simulink model "microgrid_ESS"  (R2023a)
settings: Solver=FixedStepDiscrete  StartTime=0.0  StopTime=90  FixedStep=Ts  RelTol=1e-3
PreLoadFcn:
  | %bus_ini
InitFcn:
  | %sim_param_ini
values from neighbouring files (symbols this model uses):
  Ts = 5.0E-5    [microgrid_system.sldd]
  Ts_PLC = 0.001    [microgrid_system.sldd]
undefined symbols (not defined in the file or in its folder): C, getfullname
libraries: microgridLib x37, slrealtimeutilitieslib x16, simulink x7, spsThreePhaseVIMeasurementLib x3, speedgoatlib_obsolete x3, spsPower3phInstantaneousLib x2, speedgoatlib_shared x1, spsThreePhaseSourceLib x1, spsThreePhaseFaultLib x1, spspowerguiLib x1, slrealtimetgmanagement x1
settings Model: DataDictionary=microgrid_system.sldd  SimulationMode=external  ExtModeEnableFloating=off  Creator=jlesage  LastModifiedBy=steve.liu
settings SolverCC: ConcurrentTasks=on  AlgebraicLoopSolver=TrustRegion  PositivePriorityOrder=on  AutoInsertRateTranBlk=on
settings OptimizationCC: BlockReduction=off  OptimizeBlockIOStorage=off  ReuseModelBlockBuffer=off
settings DebuggingCC: TasksWithSamePriorityMsg=none  UnconnectedInputMsg=warning  UnconnectedOutputMsg=warning  UnconnectedLineMsg=warning
settings HardwareCC: ProdBitPerLong=64  ProdLongLongMode=on  ProdHWDeviceType=Intel->x86-64 (Linux 64)
settings ModelReferenceCC: EnableRefExpFcnMdlSchedulingChecks=on
settings RTWCC: Description=Simulink Real-Time  SystemTargetFile=slrealtime.tlc  TemplateMakefile=slrealtime_default_tmf  Toolchain=Simulink Real-Time Toolchain  BuildConfiguration=Faster Runs  CodeExecutionProfiling=on  TargetLang=C++  DLArmComputeVersion=19.05

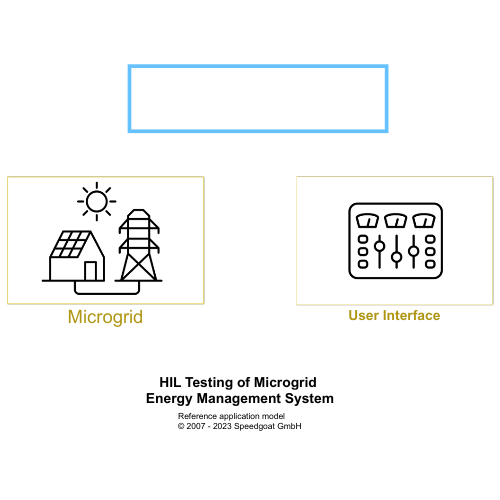
[thumbnail: Simulink's stored preview of the top-level diagram]
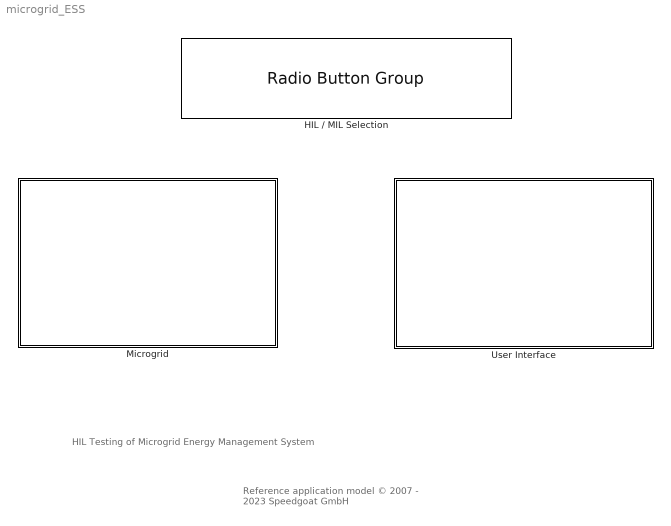
== system microgrid_ESS ==
  note: Reference application model
      | © 2007 - 2023 Speedgoat GmbH
  note: HIL Testing of Microgrid
      | Energy Management System
  HIL / MIL Selection : RadioButtonGroup  LabelPosition=Hide  SelectedLabel=Model-in-the-Loop (Desktop and real-time simulation)  ButtonGroupName=Simulation Mode
      settings: Values={{'Model-in-the-Loop (Desktop and real-time simulation)', 'Hardware-in-the-Loop'}, [0 1]}
  Microgrid : Subsystem
      mask Display: image('$imagefile'); % Use "Edit Image" on toolstrip to change.
  User Interface : Subsystem
      mask Display: image('$imagefile'); % Use "Edit Image" on toolstrip to change.

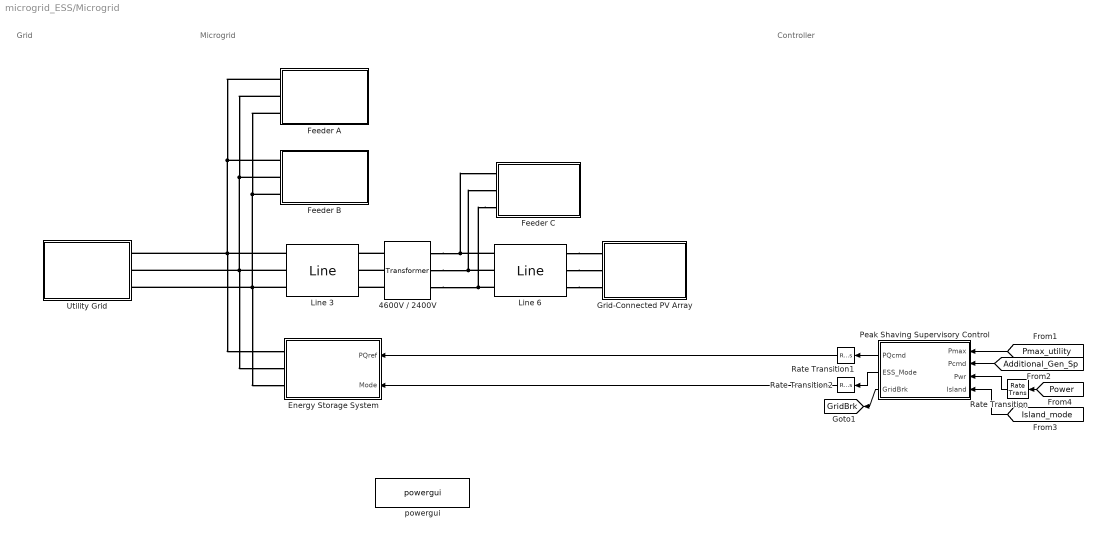
== system microgrid_ESS/Microgrid ==
  note: Microgrid
  note: Grid
  note: Controller
  4600V / 2400V : microgridLib/Transformer  kS=5000  Freq=60  Vp=4600  Vs=2400  Zperc=6.37  Ratio=3.5
  Energy Storage System : Subsystem
      settings: PortSchema="{\"entries\":[{\"content\":{\"sides\":[{\"content\":{\"connectorIds\":[\"LConn1\",\"LConn2\",\"LConn3\"]},\"type\":\"ConnectorPlacement.EquallySpacedRectSide\",\"uuid\":\"2732472e-ca9c-424c-87bd-53552b4deef9\"},{\"content\":{\"connectorIds\":[\"In1\",\"In2\"],\"side\":\"RIGHT\"},\"type\":\"ConnectorPlacement.EquallySpacedRectSide\",\"uuid\":\"774380c0-3a16-4d8f-bf4d-db561b2973b7\"},{\"content\":{\"connectorIds\":[],\"side\":\"TOP\"},\"type\":\"ConnectorPlacement.EquallySpacedRectSide\",\"uuid\":\"18303f45-8657-48d2-ba54-46513b679fcd\"}]},\"type\":\"ConnectorPlacement.EquallySpacedConnector\",\"uuid\":\"7e47473e-856d-4ee6-aecb-5fd96cc13303\"}],\"packageUris\":[\"http://schema.mathworks.com/mf0/Connector/R2020b\"],\"version\":\"1.0\"}"
      mask Display: image('$imagefile'); % Use "Edit Image" on toolstrip to change.
  Feeder A : Subsystem
      mask Display: image('$imagefile'); % Use "Edit Image" on toolstrip to change.
  Feeder B : Subsystem
      mask Display: image('$imagefile'); % Use "Edit Image" on toolstrip to change.
  Feeder C : Subsystem
      mask Display: image('$imagefile'); % Use "Edit Image" on toolstrip to change.
  Grid-Connected PV Array : Subsystem
      mask Display: image('$imagefile'); % Use "Edit Image" on toolstrip to change.
  Line 3 : microgridLib/Line   gauge=500 Kcmil  Freq=60  Length_ft=300  Ratio=3
  Line 6 : microgridLib/Line   gauge=4/0 AWG  Freq=60  Length_ft=25  Ratio=3
  Peak Shaving Supervisory Control : Subsystem  Variant=on
      mask Display: image('$imagefile'); % Use "Edit Image" on toolstrip to change.
  Rate Transition : RateTransition  OutPortSampleTime=Ts_PLC
  Rate Transition1 : RateTransition  OutPortSampleTime=Ts_Control
  Rate Transition2 : RateTransition  OutPortSampleTime=Ts_Control
  Utility Grid : Subsystem
      mask Display: image('$imagefile'); % Use "Edit Image" on toolstrip to change.
  powergui : spspowerguiLib/powergui  Priority=2  SimulationMode=Discrete  SampleTime=Ts  frequency=60  Iterations=50  frequencyindice=0  Pbase=1e6  ErrMax=0.0001  UnitsV=kV  UnitsW=MW  buscounter=6  FunctionMessages=off  echomessages=off  EnableUseOfTLC=off  CurrentSourceSwitches=off  DisableSnubberDevices=off  DisableRonSwitches=off  DisableVfSwitches=off  DisplayEquations=off  AutomaticDiscreteSolvers=off  SolverType=Tustin/Backward Euler (TBE)  Interpol=off  ExternalGateDelay=off  methode=off  Ts=0  x0status=blocks  SPID=off  SwTol=0  HookPort=off  NonlinearTolerance=1e-4  nMaxIteration=100  ContinueOnMaxIteration=off  RestoreLinks=warning  ResistiveCurrentMeasurement=off  Frange=logspace(0,3,50)  Ylog=off  Xlog=off  ShowGrid=off  save=off  variable=ZData  structure=0  ZoomFFT=on  StartTime=0.0  cycles=2  DisplayStyle=off  fundamental=60  FreqAxis=off  MaxFrequency=1000  frequencyindicesteady=1  RmsSteady=1  display=off
  tag scope: GridBrk=global
  wires:
  [Pmax_utility] -> Peak Shaving Supervisory Control/1(Pmax)
  [Additional_Gen_Sp] -> Peak Shaving Supervisory Control/2(Pcmd)
  Peak Shaving Supervisory Control/1(PQcmd) -> Rate Transition1/1
  [Island_mode] -> Peak Shaving Supervisory Control/4(Island)
  Rate Transition/1 -> Peak Shaving Supervisory Control/3(Pwr)
  Peak Shaving Supervisory Control/3(GridBrk) -> [GridBrk]
  [Power] -> Rate Transition/1
  Peak Shaving Supervisory Control/2(ESS_Mode) -> Rate Transition2/1
  Rate Transition1/1 -> Energy Storage System/1(PQref)
  Rate Transition2/1 -> Energy Storage System/2(Mode)
  connections:
  4600V / 2400V/LConn3 -- Line 3/RConn3
  Feeder C/LConn3 -- 4600V / 2400V/RConn3 -- Line 6/LConn3
  4600V / 2400V/LConn2 -- Line 3/RConn2
  Line 6/LConn2 -- 4600V / 2400V/RConn2 -- Feeder C/LConn2
  4600V / 2400V/LConn1 -- Line 3/RConn1
  Line 6/LConn1 -- 4600V / 2400V/RConn1 -- Feeder C/LConn1
  Line 3/LConn1 -- Feeder A/LConn1 -- Feeder B/LConn1 -- Utility Grid/RConn1 -- Energy Storage System/LConn1
  Line 3/LConn3 -- Feeder A/LConn3 -- Feeder B/LConn3 -- Utility Grid/RConn3 -- Energy Storage System/LConn3
  Feeder B/LConn2 -- Feeder A/LConn2 -- Utility Grid/RConn2 -- Energy Storage System/LConn2 -- Line 3/LConn2
  Line 6/RConn1 -- Grid-Connected PV Array/LConn1
  Line 6/RConn2 -- Grid-Connected PV Array/LConn2
  Line 6/RConn3 -- Grid-Connected PV Array/LConn3

== system microgrid_ESS/User Interface ==
  note: Power [W]
  note: Microgrid Peak-Shaving Control
  note: Additional Battery
      | Supply [MW]
  note: Utility Max Power
      | Setpoint [MW]
  note: Current
      | [A]
  Dashboard Scope : DashboardScope  TimeSpan=90  Ymin=-1e6  Ymax=1.5e6  ScaleAtStop=off
  Dashboard Scope1 : DashboardScope  TimeSpan=90  Ymin=-100  Ymax=100  ScaleAtStop=off
  Instrumentation : Subsystem
      mask Display: image('$imagefile'); % Use "Edit Image" on toolstrip to change.
  Knob : KnobBlock  ScaleMax=3
  Knob1 : KnobBlock  ScaleMin=-3  ScaleMax=3
  Toggle Switch : ToggleSwitchBlock  LabelPosition=Hide
      settings: Values={{'Grid Connect', 'Island'}, [0 1]}
  Toggle Switch1 : ToggleSwitchBlock  LabelPosition=Hide
      settings: Values={{'Clear', 'Cloud'}, [0 1]}

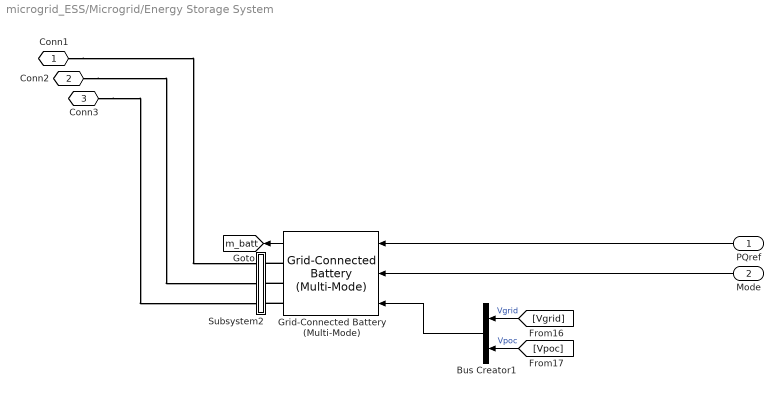
== system microgrid_ESS/Microgrid/Energy Storage System ==
  PQref : Inport
  Mode : Inport  Port=2
  Bus Creator1 : BusCreator  Inputs=2
  Grid-Connected Battery (Multi-Mode) : microgridLib/Grid-Connected Battery (Multi-Mode)  Pmod=25  Vnom_dc=480  Bcap=500  Vnom_prim=4600  Fnom=60  Ts=Ts  Ts_Control=Ts_Control
  Subsystem2 : Subsystem
  Conn1 : PMIOPort  Side=Left
  Conn2 : PMIOPort  Port=2  Side=Left
  Conn3 : PMIOPort  Port=3  Side=Left
  tag scope: m_batt=global
  wires:
  Bus Creator1/1 -> Grid-Connected Battery (Multi-Mode)/3
  Grid-Connected Battery (Multi-Mode)/1 -> [m_batt]
  [Vgrid] -> Bus Creator1/1  "Vgrid"
  [Vpoc] -> Bus Creator1/2  "Vpoc"
  PQref/1 -> Grid-Connected Battery (Multi-Mode)/1
  Mode/1 -> Grid-Connected Battery (Multi-Mode)/2
  connections:
  Grid-Connected Battery (Multi-Mode)/RConn2 -- Subsystem2/RConn2
  Grid-Connected Battery (Multi-Mode)/RConn3 -- Subsystem2/RConn3
  Grid-Connected Battery (Multi-Mode)/RConn1 -- Subsystem2/RConn1
  Conn2/RConn1 -- Subsystem2/LConn2
  Conn3/RConn1 -- Subsystem2/LConn3
  Conn1/RConn1 -- Subsystem2/LConn1

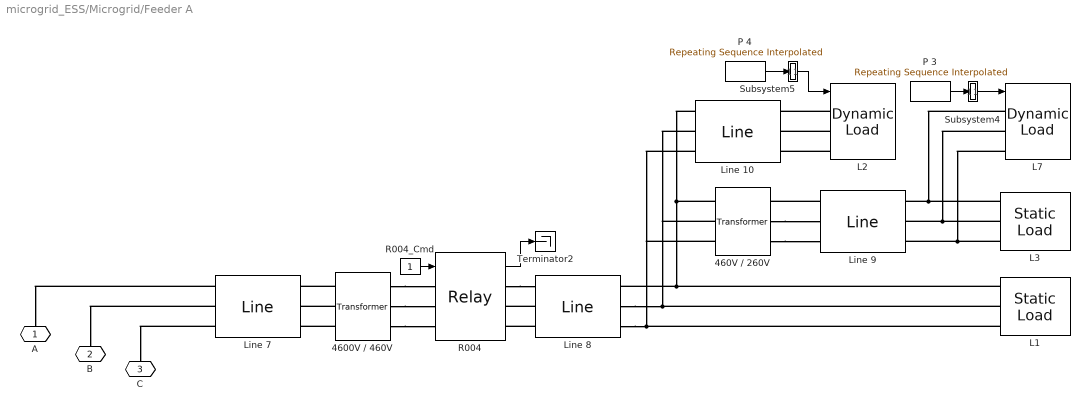
== system microgrid_ESS/Microgrid/Feeder A ==
  4600V / 460V : microgridLib/Transformer  kS=5000  Freq=60  Vp=4600  Vs=460  Zperc=5.1  Ratio=2.5
  460V / 260V : microgridLib/Transformer  kS=2000  Freq=60  Vp=460  Vs=240  Zperc=5.1  Ratio=2.5
  L1 : microgridLib/Static Load  kS=25  PF=0.9  Vrms=460  Freq=60
  L2 : microgridLib/Dynamic Load  Vrms=460  Freq=60  Ts=Ts  Tau=1e-4
  L3 : microgridLib/Static Load  kS=25  PF=1  Vrms=240  Freq=60
  L7 : microgridLib/Dynamic Load  Vrms=240  Freq=60  Ts=Ts  Tau=1e-4
  Line 10 : microgridLib/Line   gauge=3/0 AWG  Freq=60  Length_ft=50  Ratio=3
  Line 7 : microgridLib/Line   gauge=500 Kcmil  Freq=60  Length_ft=500  Ratio=3
  Line 8 : microgridLib/Line   gauge=500 Kcmil  Freq=60  Length_ft=100  Ratio=3
  Line 9 : microgridLib/Line   gauge=1/0 AWG  Freq=60  Length_ft=25  Ratio=3
  P 3 : simulink/Sources/Repeating Sequence Interpolated  OutValues=[0 -1e5 3e5 10e5 0e5 5e5 0]'/50  TimeValues=[0 5 10 25 30 45 60]'*0.2  LookUpMeth=Interpolation-Use End Values  tsamp=Ts  OutMin=[]  OutMax=[]  OutDataTypeStr=double  OutputDataTypeScalingMode=double  OutDataType=fixdt(0,8)  OutScaling=2^-10
  P 4 : simulink/Sources/Repeating Sequence Interpolated  OutValues=[0 1e5 -3e5 10e5 0e5 5e5 0]'/75  TimeValues=[0 5 10 25 30 45 60]'*0.5  LookUpMeth=Interpolation-Use End Values  tsamp=Ts  OutMin=[]  OutMax=[]  OutDataTypeStr=double  OutputDataTypeScalingMode=double  OutDataType=fixdt(0,8)  OutScaling=2^-10
  R004 : microgridLib/Relay  SystemSampleTime=-1  VariantActivationTime=update diagram  Latency=0  AutoFrameSizeCalculation=off
  R004_Cmd : Constant
  Subsystem4 : Subsystem
  Subsystem5 : Subsystem
  Terminator2 : Terminator
  A : PMIOPort  Side=Left
  B : PMIOPort  Port=2  Side=Left
  C : PMIOPort  Port=3  Side=Left
  wires:
  R004_Cmd/1 -> R004/1
  P 3/1 -> Subsystem4/1(In1)
  Subsystem4/1(Out1) -> L7/1
  P 4/1 -> Subsystem5/1(In1)
  Subsystem5/1(Out1) -> L2/1
  R004/1 -> Terminator2/1
  connections:
  Line 7/LConn2 -- B/RConn1
  Line 7/LConn3 -- C/RConn1
  Line 7/LConn1 -- A/RConn1
  4600V / 460V/RConn1 -- R004/LConn1
  4600V / 460V/LConn3 -- Line 7/RConn3
  Line 8/RConn3 -- 460V / 260V/LConn3 -- Line 10/LConn3 -- L1/LConn3
  L2/LConn1 -- Line 10/RConn1
  R004/RConn1 -- Line 8/LConn1
  4600V / 460V/RConn3 -- R004/LConn3
  Line 8/LConn3 -- R004/RConn3
  Line 8/LConn2 -- R004/RConn2
  4600V / 460V/LConn1 -- Line 7/RConn1
  Line 10/LConn1 -- 460V / 260V/LConn1 -- L1/LConn1 -- Line 8/RConn1
  Line 8/RConn2 -- 460V / 260V/LConn2 -- Line 10/LConn2 -- L1/LConn2
  4600V / 460V/LConn2 -- Line 7/RConn2
  4600V / 460V/RConn2 -- R004/LConn2
  L3/LConn3 -- L7/LConn3 -- Line 9/LConn3
  L2/LConn2 -- Line 10/RConn2
  L2/LConn3 -- Line 10/RConn3
  460V / 260V/RConn2 -- Line 9/RConn2
  Line 9/RConn1 -- 460V / 260V/RConn1
  L3/LConn1 -- L7/LConn1 -- Line 9/LConn1
  460V / 260V/RConn3 -- Line 9/RConn3
  L3/LConn2 -- L7/LConn2 -- Line 9/LConn2

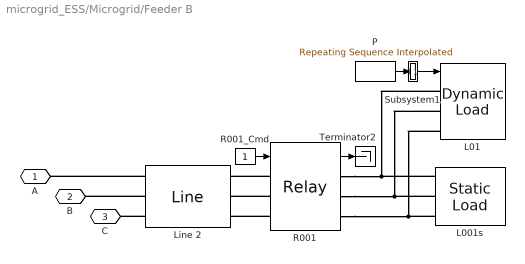
== system microgrid_ESS/Microgrid/Feeder B ==
  L001s : microgridLib/Static Load  kS=700  PF=0.99  Vrms=4600  Freq=60
  L01 : microgridLib/Dynamic Load  Vrms=4600  Freq=60  Ts=Ts  Tau=1e-4
  Line 2 : microgridLib/Line   gauge=500 Kcmil  Freq=60  Length_ft=100  Ratio=3
  "P " : simulink/Sources/Repeating Sequence Interpolated  OutValues=[0 -1e5 3e5 10e5 0e5 9e5 0 2e5 -1e5 8e5 6e5 0e5]'*0.75  TimeValues=[0 5 10 25 30 45 55 60 65 70 80 90]'  LookUpMeth=Interpolation-Use End Values  tsamp=Ts  OutMin=[]  OutMax=[]  OutDataTypeStr=double  OutputDataTypeScalingMode=double  OutDataType=fixdt(0,8)  OutScaling=2^-10
  R001 : microgridLib/Relay  SystemSampleTime=-1  VariantActivationTime=update diagram  Latency=0  AutoFrameSizeCalculation=off
  R001_Cmd : Constant
  Subsystem1 : Subsystem
  Terminator2 : Terminator
  A : PMIOPort  Side=Left
  B : PMIOPort  Port=2  Side=Left
  C : PMIOPort  Port=3  Side=Left
  wires:
  R001/1 -> Terminator2/1
  Subsystem1/1(Out1) -> L01/1
  R001_Cmd/1 -> R001/1
  "P "/1 -> Subsystem1/1(In1)
  connections:
  Line 2/LConn1 -- A/RConn1
  Line 2/LConn3 -- C/RConn1
  Line 2/LConn2 -- B/RConn1
  R001/LConn1 -- Line 2/RConn1
  R001/RConn2 -- L01/LConn2 -- L001s/LConn2
  R001/RConn1 -- L001s/LConn1 -- L01/LConn1
  R001/LConn3 -- Line 2/RConn3
  R001/RConn3 -- L01/LConn3 -- L001s/LConn3
  R001/LConn2 -- Line 2/RConn2

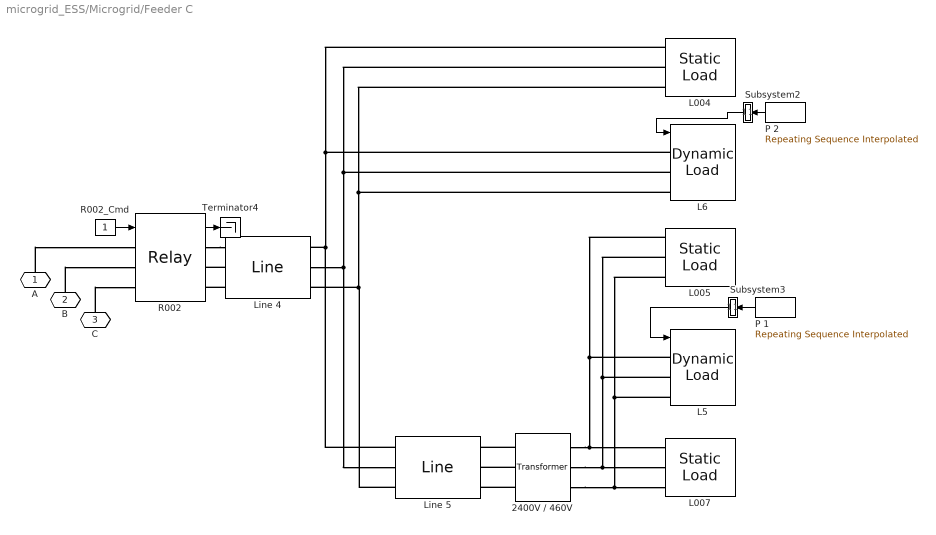
== system microgrid_ESS/Microgrid/Feeder C ==
  2400V / 460V : microgridLib/Transformer  kS=2000  Freq=60  Vp=2400  Vs=460  Zperc=5.18  Ratio=2.5
  L004 : microgridLib/Static Load  kS=25  PF=0.9  Vrms=2400  Freq=60
  L005 : microgridLib/Static Load  kS=25  PF=0.8  Vrms=460  Freq=60
  L007 : microgridLib/Static Load  kS=115  PF=0.9  Vrms=460  Freq=60
  L5 : microgridLib/Dynamic Load  Vrms=460  Freq=60  Ts=Ts  Tau=1e-4
  L6 : microgridLib/Dynamic Load  Vrms=2400  Freq=60  Ts=Ts  Tau=1e-4
  Line 4 : microgridLib/Line   gauge=500 Kcmil  Freq=60  Length_ft=100  Ratio=3
  Line 5 : microgridLib/Line   gauge=4/0 AWG  Freq=60  Length_ft=250  Ratio=3
  P 1 : simulink/Sources/Repeating Sequence Interpolated  OutValues=[0 1e5 -3e5 10e5 0e5 5e5 0]'/100  TimeValues=[0 5 10 25 30 45 60]'*0.9  LookUpMeth=Interpolation-Use End Values  tsamp=Ts  OutMin=[]  OutMax=[]  OutDataTypeStr=double  OutputDataTypeScalingMode=double  OutDataType=fixdt(0,8)  OutScaling=2^-10
  P 2 : simulink/Sources/Repeating Sequence Interpolated  OutValues=[0 -1e5 3e5 10e5 0e5 5e5 0]'/10  TimeValues=[0 5 10 25 30 45 60]'*0.1  LookUpMeth=Interpolation-Use End Values  tsamp=Ts  OutMin=[]  OutMax=[]  OutDataTypeStr=double  OutputDataTypeScalingMode=double  OutDataType=fixdt(0,8)  OutScaling=2^-10
  R002 : microgridLib/Relay  SystemSampleTime=-1  VariantActivationTime=update diagram  Latency=0  AutoFrameSizeCalculation=off
  R002_Cmd : Constant
  Subsystem2 : Subsystem
  Subsystem3 : Subsystem
  Terminator4 : Terminator
  A : PMIOPort  Side=Left
  B : PMIOPort  Port=2  Side=Left
  C : PMIOPort  Port=3  Side=Left
  wires:
  R002_Cmd/1 -> R002/1
  R002/1 -> Terminator4/1
  Subsystem3/1(Out1) -> L5/1
  Subsystem2/1(Out1) -> L6/1
  P 1/1 -> Subsystem3/1(In1)
  P 2/1 -> Subsystem2/1(In1)
  connections:
  A/RConn1 -- R002/LConn1
  B/RConn1 -- R002/LConn2
  C/RConn1 -- R002/LConn3
  Line 4/LConn3 -- R002/RConn3
  Line 5/LConn1 -- L6/LConn1 -- L004/LConn1 -- Line 4/RConn1
  2400V / 460V/LConn3 -- Line 5/RConn3
  L005/LConn2 -- L5/LConn2 -- 2400V / 460V/RConn2 -- L007/LConn2
  Line 4/LConn2 -- R002/RConn2
  2400V / 460V/LConn1 -- Line 5/RConn1
  R002/RConn1 -- Line 4/LConn1
  2400V / 460V/LConn2 -- Line 5/RConn2
  L005/LConn3 -- L5/LConn3 -- 2400V / 460V/RConn3 -- L007/LConn3
  L005/LConn1 -- L5/LConn1 -- 2400V / 460V/RConn1 -- L007/LConn1
  Line 4/RConn2 -- L6/LConn2 -- L004/LConn2 -- Line 5/LConn2
  Line 5/LConn3 -- L6/LConn3 -- L004/LConn3 -- Line 4/RConn3

== system microgrid_ESS/Microgrid/Grid-Connected PV Array ==
  Grid-Connected PV Array : microgridLib/Grid-Connected PV Array  Pmod=5  Vnom_prim=2400  Fnom=60  Ts=Ts  Ts_Control=Ts_Control
  Ir : simulink/Sources/Repeating Sequence Interpolated  OutValues=[1000 920 950 800 950 875 1000]'  TimeValues=[0 5 10 25 30 45 60]'*1.1  LookUpMeth=Interpolation-Use End Values  tsamp=Ts  OutMin=[]  OutMax=[]  OutDataTypeStr=double  OutputDataTypeScalingMode=double  OutDataType=fixdt(0,8)  OutScaling=2^-10
  Subsystem6 : Subsystem
  T : simulink/Sources/Repeating Sequence Interpolated  OutValues=[45 40 40 41 46 47 45]'  TimeValues=[0 5 10 25 30 45 60]'*1.25  LookUpMeth=Interpolation-Use End Values  tsamp=Ts  OutMin=[]  OutMax=[]  OutDataTypeStr=double  OutputDataTypeScalingMode=double  OutDataType=fixdt(0,8)  OutScaling=2^-10
  A : PMIOPort  Side=Left
  B : PMIOPort  Port=2  Side=Left
  C : PMIOPort  Port=3  Side=Left
  tag scope: m_PV=global
  wires:
  Subsystem6/1(Out1) -> Grid-Connected PV Array/1
  T/1 -> Grid-Connected PV Array/2
  Grid-Connected PV Array/1 -> [m_PV]
  Ir/1 -> Subsystem6/1(In1)
  connections:
  Grid-Connected PV Array/RConn2 -- B/RConn1
  Grid-Connected PV Array/RConn3 -- C/RConn1
  Grid-Connected PV Array/RConn1 -- A/RConn1

== system microgrid_ESS/Microgrid/Peak Shaving Supervisory Control ==
  note: 1) Add Subsystem or Model blocks as valid variant choices.
      | 2) You cannot connect blocks at this level. At simulation, connectivity is automatically
      | determined, based on the active variant and port name matching.
  Pmax : Inport
  Pcmd : Inport  Port=2
  Pwr : Inport  Port=3
  Island : Inport  Port=4
  HIL : Subsystem  VariantControl=strcmp(get_param(getfullname(Simulink.findBlocks(bdroot,'Name','SimulationSelection')),'value'),'1')
  MIL : Subsystem  VariantControl=strcmp(get_param(getfullname(Simulink.findBlocks(bdroot,'Name','SimulationSelection')),'value'),'0')
  PQcmd : Outport
  ESS_Mode : Outport  Port=2
  GridBrk : Outport  Port=3

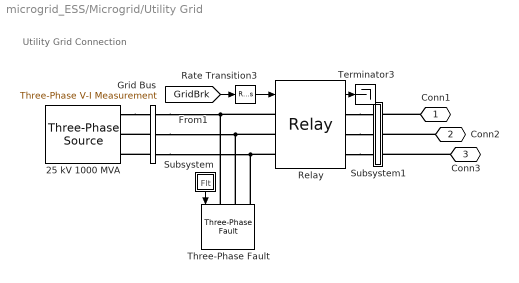
== system microgrid_ESS/Microgrid/Utility Grid ==
  note: Utility Grid Connection
  25 kV 1000 MVA : spsThreePhaseSourceLib/Three-Phase Source  InternalConnection=Yg  VoltagePhases=off  Voltage=25e3  PhaseAngle=0.34499  Voltage_phases=[25e3 25e3 25e3]/sqrt(3)  PhaseAngles_phases=[0 -120 +120]  Frequency=60  NonIdealSource=on  SpecifyImpedance=on  Resistance=25^2/1000/10  Inductance=25^2/1000/377  ShortCircuitLevel=1000e6  BaseVoltage=25e3  XRratio=10  BusType=swing  Pref=0  Qref=0  Prefabc=[10e3, 10e3, 10e3]  Qrefabc=[0, 0, 0]  Qmin=-Inf  Qmax=Inf
  Grid Bus : spsThreePhaseVIMeasurementLib/Three-Phase V-I Measurement  VoltageMeasurement=phase-to-ground  SetLabelV=on  LabelV=Vgrid  Vpu=off  VpuLL=off  CurrentMeasurement=yes  SetLabelI=on  LabelI=Igrid  Ipu=off  Pbase=100e6  Vbase=(25000)*1.00007  OutputType=Complex  PhasorSimulation=off  PSBequivalent=0
  Rate Transition3 : RateTransition  InitialCondition=1  OutPortSampleTime=Ts
  Relay : microgridLib/Relay  SystemSampleTime=-1  VariantActivationTime=update diagram  Latency=0  AutoFrameSizeCalculation=off
  Subsystem : Subsystem
  Subsystem1 : Subsystem
  Terminator3 : Terminator
  Three-Phase Fault : spsThreePhaseFaultLib/Three-Phase Fault  InitialStates=0  FaultA=on  FaultB=on  FaultC=on  GroundFault=on  SwitchTimes="[1/60  5/60]"  External=on  SwitchStatus=NaN  FaultResistance=0.01  GroundResistance=0.001  SnubberResistance=inf  SnubberCapacitance=inf  Measurements=None
  Conn1 : PMIOPort  Side=Right
  Conn2 : PMIOPort  Port=2  Side=Right
  Conn3 : PMIOPort  Port=3  Side=Right
  wires:
  [GridBrk] -> Rate Transition3/1
  Subsystem/1(Flt) -> Three-Phase Fault/1
  Rate Transition3/1 -> Relay/1
  Relay/1 -> Terminator3/1
  connections:
  Relay/LConn2 -- Grid Bus/RConn2 -- Three-Phase Fault/LConn2
  Relay/RConn1 -- Subsystem1/LConn1
  Relay/LConn3 -- Grid Bus/RConn3 -- Three-Phase Fault/LConn3
  Relay/RConn2 -- Subsystem1/LConn2
  Grid Bus/LConn3 -- 25 kV 1000 MVA/RConn3
  Grid Bus/LConn2 -- 25 kV 1000 MVA/RConn2
  Relay/RConn3 -- Subsystem1/LConn3
  Relay/LConn1 -- Grid Bus/RConn1 -- Three-Phase Fault/LConn1
  Conn3/RConn1 -- Subsystem1/RConn3
  25 kV 1000 MVA/RConn1 -- Grid Bus/LConn1
  Conn2/RConn1 -- Subsystem1/RConn2
  Conn1/RConn1 -- Subsystem1/RConn1

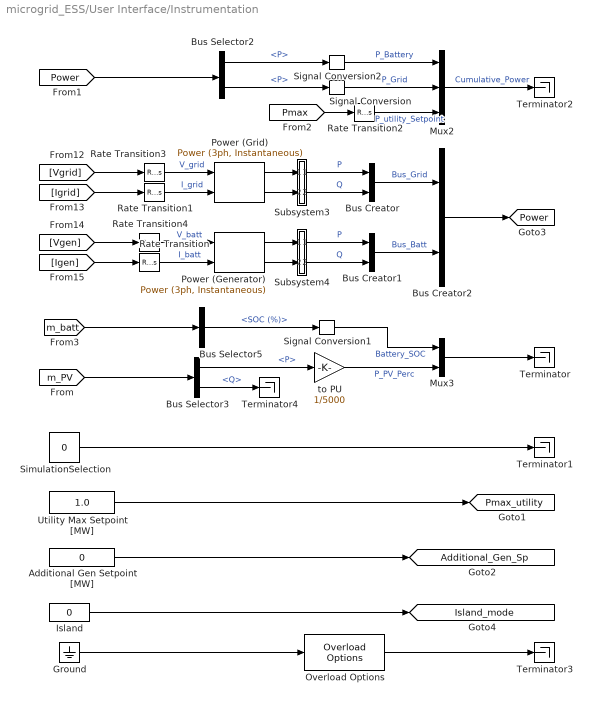
== system microgrid_ESS/User Interface/Instrumentation ==
  Additional Gen Setpoint [MW] : Constant  Value=0
  Bus Creator : BusCreator  Inputs=2  OutDataTypeStr=Bus: Grid  NonVirtualBus=on
  Bus Creator1 : BusCreator  Inputs=2  OutDataTypeStr=Bus: Batt  NonVirtualBus=on
  Bus Creator2 : BusCreator  Inputs=2  OutDataTypeStr=Bus: PowerBus  NonVirtualBus=on
  Bus Selector2 : BusSelector  OutputSignals=Bus_Batt.P,Bus_Grid.P
  Bus Selector3 : BusSelector  OutputSignals=Grid.P,Grid.Q
  Bus Selector5 : BusSelector  OutputSignals=Battery.SOC (%)
  Ground : Ground
  Island : Constant  Value=0
  Mux2 : Mux  Inputs=3
  Mux3 : Mux  Inputs=2
  Overload Options : slrealtimetgmanagement/Overload Options  startupDur=1  startupDurSrc=Tunable Parameter  maxOverload=1e6  maxOverloadSrc=Tunable Parameter  TETFlag=off
  Power (Generator) : spsPower3phInstantaneousLib/Power (3ph, Instantaneous)
  Power (Grid) : spsPower3phInstantaneousLib/Power (3ph, Instantaneous)
  Rate Transition{,1..4} (5 alike) : RateTransition  OutPortSampleTime=1e-3
  Signal Conversion : SignalConversion  OverrideOpt=off
  Signal Conversion1 : SignalConversion  OverrideOpt=off
  Signal Conversion2 : SignalConversion  OverrideOpt=off
  SimulationSelection : Constant  Value=0  OutDataTypeStr=uint8
  Subsystem3 : Subsystem
  Subsystem4 : Subsystem
  Terminator{,1..4} (5 alike) : Terminator
  Utility Max Setpoint [MW] : Constant  Value=1.0
  to PU : Gain  Gain=1/5000
  tag scope: Additional_Gen_Sp=global, Island_mode=global, Pmax_utility=global, Power=global
  wires:
  Power (Grid)/1 -> Subsystem3/1(In1)
  Bus Selector5/1 -> Signal Conversion1/1  "<SOC (%)>"
  [Vgrid] -> Rate Transition3/1
  Bus Selector3/2 -> Terminator4/1  "<Q>"
  [Power] -> Bus Selector2/1
  Subsystem3/2(Out2) -> Bus Creator/2  "Q"
  [m_PV] -> Bus Selector3/1
  Power (Grid)/2 -> Subsystem3/2(In2)
  [Igrid] -> Rate Transition1/1
  Bus Selector2/2 -> Signal Conversion/1  "<P>"
  Bus Creator1/1 -> Bus Creator2/2  "Bus_Batt"
  Bus Selector3/1 -> to PU/1  "<P>"
  Signal Conversion/1 -> Mux2/2  "P_Grid"
  Overload Options/1 -> Terminator3/1
  Subsystem4/1(Out1) -> Bus Creator1/1  "P"
  Bus Creator2/1 -> [Power]
  Mux3/1 -> Terminator/1
  [Igen] -> Rate Transition/1
  [Vgen] -> Rate Transition4/1
  Power (Generator)/2 -> Subsystem4/2(In2)
  Signal Conversion1/1 -> Mux3/1  "Battery_SOC"
  to PU/1 -> Mux3/2  "P_PV_Perc"
  [m_batt] -> Bus Selector5/1
  [Pmax] -> Rate Transition2/1
  Bus Creator/1 -> Bus Creator2/1  "Bus_Grid"
  Mux2/1 -> Terminator2/1  "Cumulative_Power"
  Ground/1 -> Overload Options/1
  SimulationSelection/1 -> Terminator1/1
  Subsystem3/1(Out1) -> Bus Creator/1  "P"
  Power (Generator)/1 -> Subsystem4/1(In1)
  Subsystem4/2(Out2) -> Bus Creator1/2  "Q"
  Bus Selector2/1 -> Signal Conversion2/1  "<P>"
  Utility Max Setpoint [MW]/1 -> [Pmax_utility]
  Additional Gen Setpoint [MW]/1 -> [Additional_Gen_Sp]
  Island/1 -> [Island_mode]
  Signal Conversion2/1 -> Mux2/1  "P_Battery"
  Rate Transition1/1 -> Power (Grid)/2  "I_grid"
  Rate Transition/1 -> Power (Generator)/2  "I_batt"
  Rate Transition2/1 -> Mux2/3  "P_utility_Setpoint"
  Rate Transition3/1 -> Power (Grid)/1  "V_grid"
  Rate Transition4/1 -> Power (Generator)/1  "V_batt"

== system microgrid_ESS/Microgrid/Energy Storage System/Subsystem2 ==
  Generator Bus : Subsystem
  Line 1 : microgridLib/Line   gauge=500 Kcmil  Freq=60  Length_ft=50  Ratio=3
  Conn1 : PMIOPort  Side=Left
  Conn2 : PMIOPort  Port=2  Side=Left
  Conn3 : PMIOPort  Port=3  Side=Left
  Conn4 : PMIOPort  Port=4  Side=Right
  Conn5 : PMIOPort  Port=5  Side=Right
  Conn6 : PMIOPort  Port=6  Side=Right
  connections:
  Line 1/LConn2 -- Conn2/RConn1
  Line 1/LConn1 -- Conn1/RConn1
  Conn4/RConn1 -- Generator Bus/LConn1
  Conn5/RConn1 -- Generator Bus/LConn2
  Conn6/RConn1 -- Generator Bus/LConn3
  Line 1/LConn3 -- Conn3/RConn1
  Line 1/RConn3 -- Generator Bus/RConn3
  Line 1/RConn2 -- Generator Bus/RConn2
  Line 1/RConn1 -- Generator Bus/RConn1

== system microgrid_ESS/Microgrid/Feeder A/Subsystem4 ==
  In1 : Inport
  Mux : Mux  Inputs=2
  Q : Constant  Value=0
  Out1 : Outport
  wires:
  Mux/1 -> Out1/1
  Q/1 -> Mux/2
  In1/1 -> Mux/1

== system microgrid_ESS/Microgrid/Feeder A/Subsystem5 ==
  In1 : Inport
  Mux : Mux  Inputs=2
  Q : Constant  Value=0
  Out1 : Outport
  wires:
  In1/1 -> Mux/1
  Q/1 -> Mux/2
  Mux/1 -> Out1/1

== system microgrid_ESS/Microgrid/Feeder B/Subsystem1 ==
  In1 : Inport
  Mux : Mux  Inputs=2
  Q : Constant  Value=0
  Out1 : Outport
  wires:
  In1/1 -> Mux/1
  Q/1 -> Mux/2
  Mux/1 -> Out1/1

== system microgrid_ESS/Microgrid/Feeder C/Subsystem2 ==
  In1 : Inport
  Mux : Mux  Inputs=2
  Q : Constant  Value=0
  Out1 : Outport
  wires:
  In1/1 -> Mux/1
  Q/1 -> Mux/2
  Mux/1 -> Out1/1

== system microgrid_ESS/Microgrid/Feeder C/Subsystem3 ==
  In1 : Inport
  Mux : Mux  Inputs=2
  Q : Constant  Value=0
  Out1 : Outport
  wires:
  In1/1 -> Mux/1
  Q/1 -> Mux/2
  Mux/1 -> Out1/1

== system microgrid_ESS/Microgrid/Grid-Connected PV Array/Subsystem6 ==
  In1 : Inport
  Constant : Constant  Value=50
  Constant1 : Constant  Value=0
  Multiport Switch : MultiPortSwitch  DataPortOrder=Zero-based contiguous  Inputs=2  zeroidx=on  SaturateOnIntegerOverflow=off  InputSameDT=off
  Out1 : Outport
  wires:
  Constant1/1 -> Multiport Switch/1
  Constant/1 -> Multiport Switch/3
  In1/1 -> Multiport Switch/2
  Multiport Switch/1 -> Out1/1

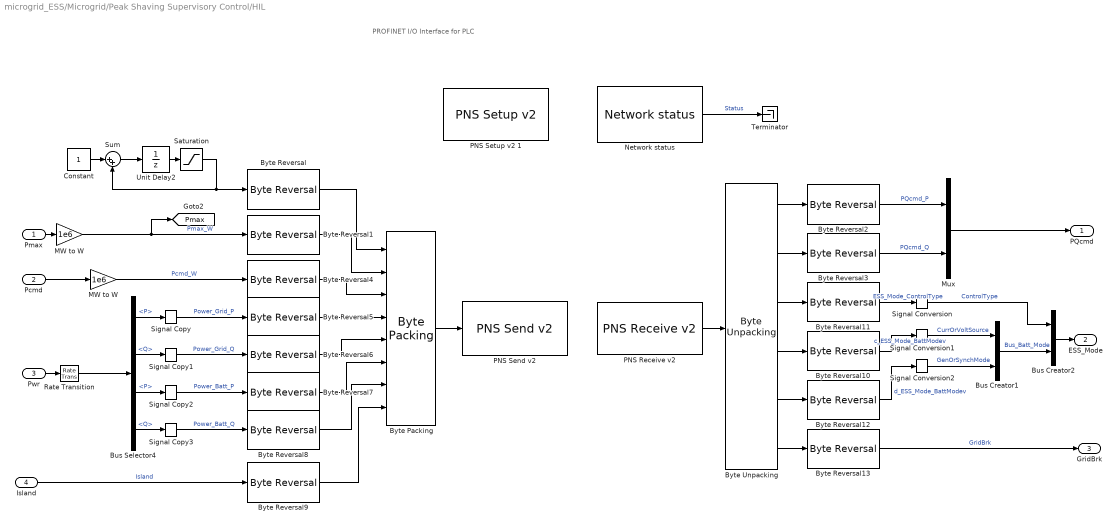
== system microgrid_ESS/Microgrid/Peak Shaving Supervisory Control/HIL ==
  note: PROFINET I/O Interface for PLC
  Pmax : Inport
  Pcmd : Inport  Port=2
  Pwr : Inport  Port=3
  Island : Inport  Port=4
  Bus Creator1 : BusCreator  Inputs=2
  Bus Creator2 : BusCreator  Inputs=2  OutDataTypeStr=Bus: ESS_Mode  NonVirtualBus=on
  Bus Selector4 : BusSelector  OutputSignals=Bus_Grid.P,Bus_Grid.Q,Bus_Batt.P,Bus_Batt.Q
  Byte Packing : slrealtimeutilitieslib/Byte Packing  MaskPackedDataType=uint8  MaskUnpackedDataTypes={'uint32','double','double','double','double','double','double','double'}  MaskAlignment=1
  Byte Reversal{,1..13} (14 alike) : slrealtimeutilitieslib/Byte Reversal  numInp=1
  Byte Unpacking : slrealtimeutilitieslib/Byte Unpacking  MaskUnpackedDataTypes={'double','double','double','double','double','double'}  MaskUnpackedDataSizes={[1],[1],[1],[1],[1],[1]}  MaskAlignment=1
  Constant : Constant  OutDataTypeStr=uint32
  MW to W : Gain  Gain=1e6
  "MW to W " : Gain  Gain=1e6
  Mux : Mux  Inputs=2
  Network status : speedgoatlib_shared/IO75X/Network status  id=2  get_status=on  set_status=off  timeout=0.01  ts=-1
  "PNS Receive v2 " : speedgoatlib_obsolete/IO752/PNS Receive v2   id=2  portType=1 port with n element vector of type UINT8  inputOutput=48  sampleTime=-1
  "PNS Send v2 " : speedgoatlib_obsolete/IO752/PNS Send v2   id=2  portType=1 port with n element vector of type UINT8  inputOutput=60  sampleTime=-1
  PNS Setup v2 1 : speedgoatlib_obsolete/IO752/PNS Setup v2   id=2  driveLetter=C:  configurationMode=Configuration file  mode=Polling mode  pciSlot=[10,6]  quantityOfAcyclicObjects=0  qtyMods=[2,0,0]  busStartup=Automatic  stationName='cifxrepns'  vendorId=hex2dec('011E')  deviceId=hex2dec('0103')  objId=1  pnModuleConfig=[]  parRecordConfigRaw={}  parRecordConfig=0  parRecordDefaults=0  RecordSuccess=on  protocol=IO752  firmware=PROFINET Device  blockVersion=3  parModuleType=IO752
  Rate Transition : RateTransition  OutPortSampleTime=Ts_PLC
  Saturation : Saturate  UpperLimit=1  LowerLimit=0  OutDataTypeStr=uint32
  Signal Conversion : SignalConversion  OverrideOpt=off
  Signal Conversion1 : SignalConversion  OverrideOpt=off
  Signal Conversion2 : SignalConversion  OverrideOpt=off
  Signal Copy{,1..3} (4 alike) : SignalConversion  OverrideOpt=off
  Sum : Sum  Inputs=|++
  Terminator : Terminator
  Unit Delay2 : UnitDelay  SampleTime=-1  HasFrameUpgradeWarning=on
  PQcmd : Outport  SampleTime=Ts_PLC
  ESS_Mode : Outport  Port=2  SampleTime=Ts_PLC
  GridBrk : Outport  Port=3  SampleTime=Ts_PLC
  tag scope: Pmax=global
  wires:
  Rate Transition/1 -> Bus Selector4/1
  Pcmd/1 -> "MW to W "/1
  Pmax/1 -> MW to W/1
  Pwr/1 -> Rate Transition/1
  Signal Conversion/1 -> Bus Creator2/1  "ControlType"
  Signal Conversion1/1 -> Bus Creator1/1  "CurrOrVoltSource"
  Signal Conversion2/1 -> Bus Creator1/2  "GenOrSynchMode"
  Bus Creator1/1 -> Bus Creator2/2  "Bus_Batt_Mode"
  Bus Creator2/1 -> ESS_Mode/1
  Mux/1 -> PQcmd/1
  Sum/1 -> Unit Delay2/1
  Constant/1 -> Sum/1
  Saturation/1 -> Sum/2, Byte Reversal/1
  Unit Delay2/1 -> Saturation/1
  MW to W/1 -> [Pmax], Byte Reversal1/1  "Pmax_W"
  "MW to W "/1 -> Byte Reversal4/1  "Pcmd_W"
  Bus Selector4/1 -> Signal Copy/1  "<P>"
  Bus Selector4/2 -> Signal Copy1/1  "<Q>"
  Bus Selector4/3 -> Signal Copy2/1  "<P>"
  Bus Selector4/4 -> Signal Copy3/1  "<Q>"
  Byte Unpacking/4 -> Byte Reversal10/1
  Byte Reversal13/1 -> GridBrk/1  "GridBrk"
  Byte Reversal1/1 -> Byte Packing/2
  Byte Unpacking/3 -> Byte Reversal11/1
  Byte Reversal9/1 -> Byte Packing/8
  Byte Unpacking/1 -> Byte Reversal2/1
  Byte Unpacking/6 -> Byte Reversal13/1
  Byte Reversal12/1 -> Signal Conversion2/1  "d_ESS_Mode_BattModev"
  Byte Reversal2/1 -> Mux/1  "PQcmd_P"
  Byte Unpacking/2 -> Byte Reversal3/1
  Byte Reversal3/1 -> Mux/2  "PQcmd_Q"
  Byte Reversal10/1 -> Signal Conversion1/1  "c_ESS_Mode_BattModev"
  Island/1 -> Byte Reversal9/1  "Island"
  Byte Reversal4/1 -> Byte Packing/3
  Byte Reversal5/1 -> Byte Packing/4
  Byte Unpacking/5 -> Byte Reversal12/1
  Signal Copy1/1 -> Byte Reversal6/1  "Power_Grid_Q"
  "PNS Receive v2 "/1 -> Byte Unpacking/1
  Byte Reversal/1 -> Byte Packing/1
  Byte Reversal11/1 -> Signal Conversion/1  "ESS_Mode_ControlType"
  Signal Copy3/1 -> Byte Reversal8/1  "Power_Batt_Q"
  Byte Reversal6/1 -> Byte Packing/5
  Byte Reversal7/1 -> Byte Packing/6
  Byte Packing/1 -> "PNS Send v2 "/1
  Byte Reversal8/1 -> Byte Packing/7
  Signal Copy2/1 -> Byte Reversal7/1  "Power_Batt_P"
  Network status/1 -> Terminator/1  "Status"
  Signal Copy/1 -> Byte Reversal5/1  "Power_Grid_P"

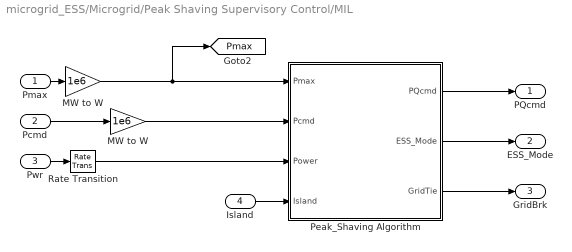
== system microgrid_ESS/Microgrid/Peak Shaving Supervisory Control/MIL ==
  Pmax : Inport
  Pcmd : Inport  Port=2
  Pwr : Inport  Port=3
  Island : Inport  Port=4
  MW to W : Gain  Gain=1e6
  "MW to W " : Gain  Gain=1e6
  Peak_Shaving Algorithm : Stateflow chart  TreatAsAtomicUnit=on  SystemSampleTime=Ts_PLC
  Rate Transition : RateTransition  OutPortSampleTime=Ts_PLC
  PQcmd : Outport  SampleTime=Ts_PLC
  ESS_Mode : Outport  Port=2  SampleTime=Ts_PLC
  GridBrk : Outport  Port=3  SampleTime=Ts_PLC
  tag scope: Pmax=global
  wires:
  Rate Transition/1 -> Peak_Shaving Algorithm/3(Power)
  Pcmd/1 -> "MW to W "/1
  Pmax/1 -> MW to W/1
  Peak_Shaving Algorithm/1(PQcmd) -> PQcmd/1
  Pwr/1 -> Rate Transition/1
  "MW to W "/1 -> Peak_Shaving Algorithm/2(Pcmd)
  MW to W/1 -> [Pmax], Peak_Shaving Algorithm/1(Pmax)
  Peak_Shaving Algorithm/3(GridTie) -> GridBrk/1
  Peak_Shaving Algorithm/2(ESS_Mode) -> ESS_Mode/1
  Island/1 -> Peak_Shaving Algorithm/4(Island)

== system microgrid_ESS/Microgrid/Utility Grid/Subsystem ==
  Fault : Constant  Value=0
  Triggered Subsystem : Subsystem  TreatAsAtomicUnit=on
  Flt : Outport
  wires:
  Fault/1 -> Triggered Subsystem/Enable
  Triggered Subsystem/1(Out1) -> Flt/1

== system microgrid_ESS/Microgrid/Utility Grid/Subsystem1 ==
  "25 kV / 4160V " : microgridLib/Transformer  kS=6000  Freq=60  Vp=25e3  Vs=4600  Zperc=5.18  Ratio=2.5
  Grid Bus1 : spsThreePhaseVIMeasurementLib/Three-Phase V-I Measurement  VoltageMeasurement=phase-to-ground  SetLabelV=on  LabelV=Vpoc  Vpu=off  VpuLL=off  CurrentMeasurement=yes  SetLabelI=on  LabelI=Ipoc  Ipu=off  Pbase=100e6  Vbase=(25000)*1.00007  OutputType=Complex  PhasorSimulation=off  PSBequivalent=0
  "Line " : microgridLib/Line   gauge=500 Kcmil  Freq=60  Length_ft=100  Ratio=3
  Conn1 : PMIOPort  Side=Left
  Conn2 : PMIOPort  Port=2  Side=Right
  Conn3 : PMIOPort  Port=3  Side=Left
  Conn4 : PMIOPort  Port=4  Side=Right
  Conn5 : PMIOPort  Port=5  Side=Left
  Conn6 : PMIOPort  Port=6  Side=Right
  connections:
  Conn4/RConn1 -- "Line "/RConn2
  Conn6/RConn1 -- "Line "/RConn3
  Conn2/RConn1 -- "Line "/RConn1
  Conn3/RConn1 -- Grid Bus1/LConn2
  Conn1/RConn1 -- Grid Bus1/LConn1
  Conn5/RConn1 -- Grid Bus1/LConn3
  "Line "/LConn2 -- "25 kV / 4160V "/RConn2
  Grid Bus1/RConn1 -- "25 kV / 4160V "/LConn1
  Grid Bus1/RConn3 -- "25 kV / 4160V "/LConn3
  "Line "/LConn1 -- "25 kV / 4160V "/RConn1
  "Line "/LConn3 -- "25 kV / 4160V "/RConn3
  Grid Bus1/RConn2 -- "25 kV / 4160V "/LConn2

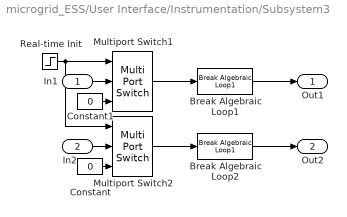
== system microgrid_ESS/User Interface/Instrumentation/Subsystem3 ==
  In1 : Inport
  In2 : Inport  Port=2
  Break Algebraic Loop1 : microgridLib/Dynamic Load/Calculate Current/Break Algebraic Loop1  Tau=0.01  Ts=Ts
  Break Algebraic Loop2 : microgridLib/Dynamic Load/Calculate Current/Break Algebraic Loop1  Tau=0.01  Ts=Ts
  Constant : Constant  Value=0
  Constant1 : Constant  Value=0
  Multiport Switch1 : MultiPortSwitch  DataPortOrder=Zero-based contiguous  Inputs=2  zeroidx=on  SaturateOnIntegerOverflow=off  InputSameDT=off
  Multiport Switch2 : MultiPortSwitch  DataPortOrder=Zero-based contiguous  Inputs=2  zeroidx=on  SaturateOnIntegerOverflow=off  InputSameDT=off
  Real-time Init : Step  Time=2  Before=1  After=0  SampleTime=Ts
  Out1 : Outport
  Out2 : Outport  Port=2
  wires:
  Real-time Init/1 -> Multiport Switch1/1, Multiport Switch2/1
  Constant1/1 -> Multiport Switch1/3
  Constant/1 -> Multiport Switch2/3
  Multiport Switch1/1 -> Break Algebraic Loop1/1
  In2/1 -> Multiport Switch2/2
  In1/1 -> Multiport Switch1/2
  Multiport Switch2/1 -> Break Algebraic Loop2/1
  Break Algebraic Loop1/1 -> Out1/1
  Break Algebraic Loop2/1 -> Out2/1

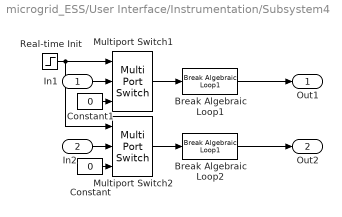
== system microgrid_ESS/User Interface/Instrumentation/Subsystem4 ==
  In1 : Inport
  In2 : Inport  Port=2
  Break Algebraic Loop1 : microgridLib/Dynamic Load/Calculate Current/Break Algebraic Loop1  Tau=0.01  Ts=Ts
  Break Algebraic Loop2 : microgridLib/Dynamic Load/Calculate Current/Break Algebraic Loop1  Tau=0.01  Ts=Ts
  Constant : Constant  Value=0
  Constant1 : Constant  Value=0
  Multiport Switch1 : MultiPortSwitch  DataPortOrder=Zero-based contiguous  Inputs=2  zeroidx=on  SaturateOnIntegerOverflow=off  InputSameDT=off
  Multiport Switch2 : MultiPortSwitch  DataPortOrder=Zero-based contiguous  Inputs=2  zeroidx=on  SaturateOnIntegerOverflow=off  InputSameDT=off
  Real-time Init : Step  Time=2  Before=1  After=0  SampleTime=Ts
  Out1 : Outport
  Out2 : Outport  Port=2
  wires:
  Multiport Switch2/1 -> Break Algebraic Loop2/1
  In1/1 -> Multiport Switch1/2
  In2/1 -> Multiport Switch2/2
  Multiport Switch1/1 -> Break Algebraic Loop1/1
  Constant/1 -> Multiport Switch2/3
  Constant1/1 -> Multiport Switch1/3
  Real-time Init/1 -> Multiport Switch2/1, Multiport Switch1/1
  Break Algebraic Loop1/1 -> Out1/1
  Break Algebraic Loop2/1 -> Out2/1

== system microgrid_ESS/Microgrid/Energy Storage System/Subsystem2/Generator Bus ==
  Grid Bus1 : spsThreePhaseVIMeasurementLib/Three-Phase V-I Measurement  VoltageMeasurement=phase-to-ground  SetLabelV=on  LabelV=Vgen  Vpu=off  VpuLL=off  CurrentMeasurement=yes  SetLabelI=on  LabelI=Igen  Ipu=off  Pbase=100e6  Vbase=(25000)*1.00007  OutputType=Complex  PhasorSimulation=off  PSBequivalent=0
  A : PMIOPort  Side=Left
  a : PMIOPort  Port=2  Side=Right
  B : PMIOPort  Port=3  Side=Left
  b : PMIOPort  Port=4  Side=Right
  C : PMIOPort  Port=5  Side=Left
  c : PMIOPort  Port=6  Side=Right
  connections:
  Grid Bus1/RConn1 -- a/RConn1
  Grid Bus1/RConn2 -- b/RConn1
  Grid Bus1/RConn3 -- c/RConn1
  C/RConn1 -- Grid Bus1/LConn3
  B/RConn1 -- Grid Bus1/LConn2
  A/RConn1 -- Grid Bus1/LConn1

== system microgrid_ESS/Microgrid/Utility Grid/Subsystem/Triggered Subsystem ==
  Enable : EnablePort  StatesWhenEnabling=reset
  Constant : Constant  Value=0
  Delay : Delay  DelayLength=round(1.05*Ts_PLC/Ts)  InitialCondition=1
  Out1 : Outport  InitialOutput=0
  wires:
  Delay/1 -> Out1/1
  Constant/1 -> Delay/1

== stateflow chart microgrid_ESS/Microgrid/Peak Shaving Supervisory Control/MIL/Peak_Shaving Algorithm ==
  state ESS_Control [parallel]
    during:
    P_Excess = Power.Bus_Grid.P + Power.Bus_Batt.P + Pcmd - Pmax;
    P_Max = genMax - Power.Bus_Batt.P;
    settings: executionOrder=1
    state GridConnected
      entry,during:
      ESS_Mode.ControlType = 0; %PQ Mode
      ESS_Mode.Bus_Batt_Mode.CurrOrVoltSource = 0; %Current Source
      isIsland = 0;
      state PeakShaving
        state MaxLocalGeneration
          during:
          PQcmd = [P_Max;0];
        state LoadFollowing
          during:
          PQcmd = [P_Excess;0];
        (default) -> LoadFollowing
        MaxLocalGeneration -> LoadFollowing : [Power.Bus_Batt.P < 0.95*genMax]
        LoadFollowing -> MaxLocalGeneration : [Power.Bus_Batt.P > genMax]
      state Nominal
        entry,during:
        PQcmd = [Pcmd;0];
      Nominal -> PeakShaving : [Power.Bus_Grid.P + Pcmd ...
          |  > Pmax]
      PeakShaving -> Nominal : [Power.Bus_Batt.P < 0 ...
          | && after(1,sec)]
      (default) -> Nominal
    state PrepareToIsland
      entry,during:
      PQcmd = [Power.Bus_Grid.P + Power.Bus_Batt.P + Pcmd; 0];
    state Islanded
      during:
      ESS_Mode.Bus_Batt_Mode.CurrOrVoltSource = 1; %Voltage Source
      ESS_Mode.Bus_Batt_Mode.GenOrSynchMode = 0; % No synch
      ESS_Mode.ControlType = 2; %No Current Control
    state Synchronize
      entry,during:
      ESS_Mode.Bus_Batt_Mode.CurrOrVoltSource = 1; %Voltage Source
      ESS_Mode.Bus_Batt_Mode.GenOrSynchMode = 1; % Synchronize
    (default) -> GridConnected
    GridConnected -> PrepareToIsland : [Island == 1]
    ESS_Control.Synchronize -> GridConnected : Reconnect
    PrepareToIsland -> ESS_Control.Islanded : [Power.Bus_Grid.P < 100]{isIsland = 1;}
    ESS_Control.Islanded -> ESS_Control.Synchronize : Synchronize
  state GridBreakerLogic [parallel]
    settings: executionOrder=2
    state Islanded
      during:
      GridTie = 0;
    state GridTied
      entry,during:
      GridTie = 1;
    state Reconnect
      entry,during:
      GridTie = 1;
      isIsland = 0;
    state Synchronize
    (default) -> GridTied
    GridTied -> GridBreakerLogic.Islanded : [isIsland == 1]
    Reconnect -> GridTied : [after(1,sec)] {send(Reconnect,ESS_Control)}
    GridBreakerLogic.Islanded -> GridBreakerLogic.Synchronize : [after(1,sec) && Island == 0] {send(Synchronize,ESS_Control)}
    GridBreakerLogic.Synchronize -> Reconnect : [after(2,sec)]
  data: Pmax input; genMax parameter; Pcmd input; Power input Bus: PowerBus; PQcmd output; ESS_Mode output Bus: ESS_Mode =0; GridTie output; P_Excess local; P_Max local; Island input; isIsland local
  events: Reconnect local FUNCTION_CALL_EVENT; Synchronize local FUNCTION_CALL_EVENT
